simulink model "Model2"  (R2023b)
settings: Solver=ode4  StartTime=0.0  StopTime=50  FixedStep=0.01  RelTol=1e-3
values from neighbouring files (symbols this model uses):
  ARM_P_PID = [10 0 20]*0.1    [Single_ARM_Monte.m]    (also in main_starter.m)
  ARM_T_PID = [100 0 0]    [Single_ARM_Monte.m]    (also in main_starter.m)
  ARM_V_PID = [10 0 5]*0.1    [Single_ARM_Monte.m]    (also in main_starter.m)
  D = sqrt(px*px + py*py)    [test2.m]
  D_Joint0_angle0 = 45    [Single_ARM_Monte.m]    (also in main_starter.m)
  D_Joint0_angle1 = 0    [Single_ARM_Monte.m]    (also in main_starter.m)
  D_Joint0_angle2 = 0    [Single_ARM_Monte.m]    (also in main_starter.m)
  D_Joint0_rate0 = 0    [Single_ARM_Monte.m]    (also in main_starter.m)
  D_Joint0_rate1 = 0    [Single_ARM_Monte.m]    (also in main_starter.m)
  D_Joint0_rate2 = 0    [Single_ARM_Monte.m]    (also in main_starter.m)
  Joint_Motor_Mass = 23    [Single_ARM_Monte.m]    (also in main_starter.m)
  L_Joint0_angle0 = 45    [Single_ARM_Monte.m]    (also in main_starter.m)
  L_Joint0_angle1 = 0    [Single_ARM_Monte.m]    (also in main_starter.m)
  L_Joint0_angle2 = 0    [Single_ARM_Monte.m]    (also in main_starter.m)
  L_Joint0_rate0 = 0    [Single_ARM_Monte.m]    (also in main_starter.m)
  L_Joint0_rate1 = 0    [Single_ARM_Monte.m]    (also in main_starter.m)
  L_Joint0_rate2 = 0    [Single_ARM_Monte.m]    (also in main_starter.m)
  L_Joint_Offset = [ ... (first row only)    [Single_ARM_Monte.m]    (also in main_starter.m)
  Link1_Mass = 11    [Single_ARM_Monte.m]    (also in main_starter.m)
  Link2_Mass = 15.6    [Single_ARM_Monte.m]    (also in main_starter.m)
  Link3_Mass = 11    [Single_ARM_Monte.m]    (also in main_starter.m)
  Motor_transfer_Den = [1 100]    [Single_ARM_Monte.m]    (also in main_starter.m)
  Motor_transfer_Num = [100]    [Single_ARM_Monte.m]    (also in main_starter.m)
  PID_dt = 0.01    [Single_ARM_Monte.m]    (also in main_starter.m)
  R_Joint0_angle0 = 45    [Single_ARM_Monte.m]    (also in main_starter.m)
  R_Joint0_angle1 = 0    [Single_ARM_Monte.m]    (also in main_starter.m)
  R_Joint0_angle2 = 0    [Single_ARM_Monte.m]    (also in main_starter.m)
  R_Joint0_rate0 = 0    [Single_ARM_Monte.m]    (also in main_starter.m)
  R_Joint0_rate1 = 0    [Single_ARM_Monte.m]    (also in main_starter.m)
  R_Joint0_rate2 = 0    [Single_ARM_Monte.m]    (also in main_starter.m)
  RW_Att_D = 0.5    [Single_ARM_Monte.m]    (also in main_starter.m)
  RW_Att_I = 0.2    [Single_ARM_Monte.m]    (also in main_starter.m)
  RW_Att_P = 0.1    [Single_ARM_Monte.m]    (also in main_starter.m)
  RW_Mass = 100    [Single_ARM_Monte.m]    (also in main_starter.m)
  S_Body_Mass = 5    [Single_ARM_Monte.m]    (also in main_starter.m)
  S_init_pos = [0 0 0]'    [Single_ARM_Monte.m]    (also in main_starter.m)
  S_init_vel = [0 0 0]'    [Single_ARM_Monte.m]    (also in main_starter.m)
  T_Body_Mass = 4    [Single_ARM_Monte.m]    (also in main_starter.m)
  T_init_pos = [T_init_pos_list(i,1) T_init_pos_list(i,2) 0]'    [Single_ARM_Monte.m]    (also in main_starter.m = [0.3 0 0]')
  T_init_vel = [0 0 0]'    [Single_ARM_Monte.m]    (also in main_starter.m)
  Torq_mea_transfer_Den = [1 5]    [Single_ARM_Monte.m]    (also in main_starter.m)
  Torq_mea_transfer_Num = [5]    [Single_ARM_Monte.m]    (also in main_starter.m)
  U_Joint0_angle0 = 45    [Single_ARM_Monte.m]    (also in main_starter.m)
  U_Joint0_angle1 = 0    [Single_ARM_Monte.m]    (also in main_starter.m)
  U_Joint0_angle2 = 0    [Single_ARM_Monte.m]    (also in main_starter.m)
  U_Joint0_rate0 = 0    [Single_ARM_Monte.m]    (also in main_starter.m)
  U_Joint0_rate1 = 0    [Single_ARM_Monte.m]    (also in main_starter.m)
  U_Joint0_rate2 = 0    [Single_ARM_Monte.m]    (also in main_starter.m)
undefined symbols (not defined in the file or in its folder): X, Y, Z
libraries: nesl_utility x315, sm_lib x281, simulink_extras x48, sharedtransform x25, aerolibutil x4
(part 8 of 12)

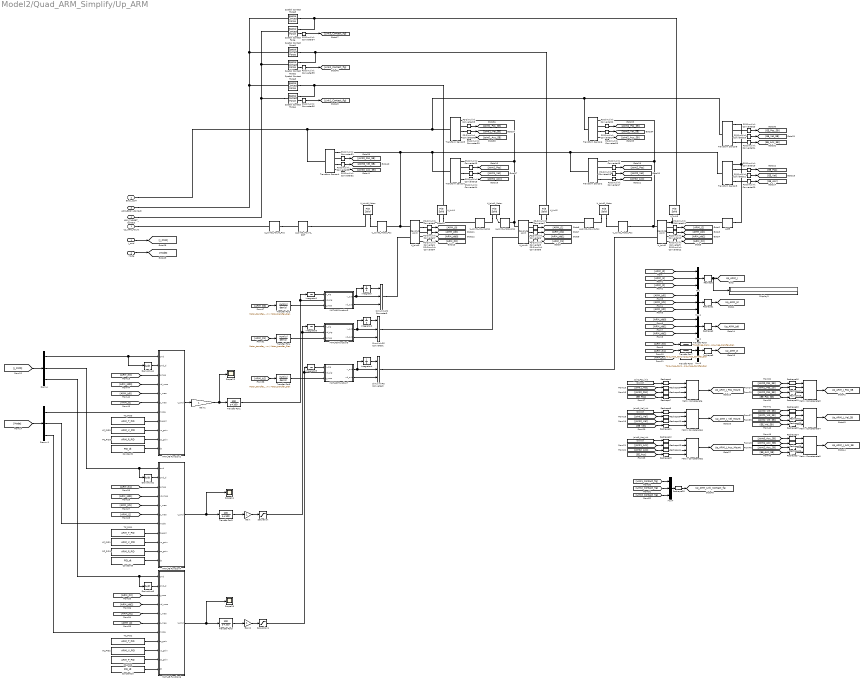
== system Model2/Quad_ARM_Simplify/Up_ARM ==
  J_cmd : Inport
  Mode : Inport  Port=2
  Constant10 : Constant  Value=PID_dt
  Constant2 : Constant  Value=PID_dt
  Constant9 : Constant  Value=PID_dt
  Demux : Demux  Outputs=3
  Demux1 : Demux  Outputs=3
  Derivative1 : Derivative
  Derivative2 : Derivative
  Derivative3 : Derivative
  Display3 : Display
  Gain : Gain
  Gain1 : Gain
  Gain2 : Gain
  Integrator : Integrator  InitialCondition=-U_Joint0_angle0*(pi/180)
  Integrator1 : Integrator  InitialCondition=-U_Joint0_rate0*(pi/180)
  Integrator2 : Integrator  InitialCondition=-U_Joint0_angle1*(pi/180)
  Integrator3 : Integrator  InitialCondition=-U_Joint0_rate1*(pi/180)
  Integrator4 : Integrator  InitialCondition=-U_Joint0_angle2*(pi/180)
  Integrator5 : Integrator  InitialCondition=-U_Joint0_rate2*(pi/180)
  Joint0_Acc_init : Constant  Value=[0 0 0]'
  Joint0_Vel_init : Constant  Value=[0 0 0]'
  Joint_Pos_init : Constant  Value=[0 0 0]'
  MATLAB Function2 : MATLAB Function  TreatAsAtomicUnit=on
  MATLAB Function3 : MATLAB Function  TreatAsAtomicUnit=on
  MATLAB Function4 : MATLAB Function  TreatAsAtomicUnit=on
  MATLAB Function5 : MATLAB Function  TreatAsAtomicUnit=on
  MATLAB Function6 : MATLAB Function  TreatAsAtomicUnit=on
  MATLAB Function7 : MATLAB Function  TreatAsAtomicUnit=on
  Matrix Concatenate{,1..5} (6 alike) : Concatenate  NumInputs=4  Mode=Multidimensional array  ConcatenateDimension=2
  Mux{,1..4} (5 alike) : Mux  Inputs=3
  PC_PID1 : Constant  Value=ARM_P_PID
  PC_PID2 : Constant  Value=ARM_P_PID
  PC_PID3 : Constant  Value=ARM_P_PID
  PS-Simulink Converter{1..36} (36 alike) : nesl_utility/PS-Simulink Converter  PhysicalDomain=network_engine_domain  SubClassName=ps_output  LeftPortType=input  RightPortType=output  PseudoPeriodic=off  Frequencies=[]  VectorFormat=inherit  Unit=inherit  AffineConversion=off
  Reshape{,1..28} (29 alike) : Reshape  OutputDimensionality=Column vector (2-D)
  Saturation : Saturate  UpperLimit=2  LowerLimit=-2
  Saturation1 : Saturate  UpperLimit=2  LowerLimit=-2
  Scope11 : Scope
  Scope13 : Scope
  Scope15 : Scope
  Simulink-PS Converter1 : nesl_utility/Simulink-PS Converter  PhysicalDomain=network_engine_domain  SubClassName=ps_input  LeftPortType=input  RightPortType=output  PseudoPeriodic=off  Frequencies=[]  NoiseDistribution=none  NoiseParameters=[]  Unit=1  AffineConversion=off  FilteringAndDerivatives=provide  SimscapeFilterOrder=1  InputFilterTimeConstant=0.001  UdotUserProvided=2
  Simulink-PS Converter2 : nesl_utility/Simulink-PS Converter  PhysicalDomain=network_engine_domain  SubClassName=ps_input  LeftPortType=input  RightPortType=output  PseudoPeriodic=off  Frequencies=[]  NoiseDistribution=none  NoiseParameters=[]  Unit=1  AffineConversion=off  FilteringAndDerivatives=provide  SimscapeFilterOrder=1  InputFilterTimeConstant=0.001  UdotUserProvided=2
  Simulink-PS Converter9 : nesl_utility/Simulink-PS Converter  PhysicalDomain=network_engine_domain  SubClassName=ps_input  LeftPortType=input  RightPortType=output  PseudoPeriodic=off  Frequencies=[]  NoiseDistribution=none  NoiseParameters=[]  Unit=1  AffineConversion=off  FilteringAndDerivatives=provide  SimscapeFilterOrder=1  InputFilterTimeConstant=0.001  UdotUserProvided=2
  Spatial Contact Force : sm_lib/Forces and Torques/Spatial Contact Force  SenseContactBaseRotation=off  SenseContactBaseTranslation=off  CoefficientOfDynamicFriction=L2T_DF  CoefficientOfStaticFriction=L2T_SF  NormalDamping=L32T_Damping  NormalDampingUnits=N/(m/s)  SenseContactSignal=on  NormalStiffness=L32T_Siffness  NormalStiffnessUnits=N/m  FrictionalCriticalVelocity=L2T_CV  FrictionalCriticalVelocityUnits=m/s  ZeroCrossDetectContactStartAndEnd=off  SenseContactFollowerRotation=off  SenseContactFollowerTranslation=off  FrictionType=SmoothStickSlip  SenseFrictionalForceMagnitude=off  SenseNormalForceMagnitude=off  NormalForceType=SmoothSpringDamper  SenseNormalVelocity=off  SensePenetrationDepth=off  SenseSeparationDistance=off  SenseTangentialVelocity=off  NormalTransitionRegionWidth=L32T_TRW  NormalTransitionRegionWidthUnits=m
  Spatial Contact Force1 : sm_lib/Forces and Torques/Spatial Contact Force  SenseContactBaseRotation=off  SenseContactBaseTranslation=off  CoefficientOfDynamicFriction=L2B_DF  CoefficientOfStaticFriction=L2B_SF  NormalDamping=L22B_Damping  NormalDampingUnits=N/(m/s)  SenseContactSignal=off  NormalStiffness=L22B_Stiffness  NormalStiffnessUnits=N/m  FrictionalCriticalVelocity=L2B_CV  FrictionalCriticalVelocityUnits=m/s  ZeroCrossDetectContactStartAndEnd=off  SenseContactFollowerRotation=off  SenseContactFollowerTranslation=off  FrictionType=SmoothStickSlip  SenseFrictionalForceMagnitude=off  SenseNormalForceMagnitude=off  NormalForceType=SmoothSpringDamper  SenseNormalVelocity=off  SensePenetrationDepth=off  SenseSeparationDistance=off  SenseTangentialVelocity=off  NormalTransitionRegionWidth=L22B_TRW  NormalTransitionRegionWidthUnits=m
  Spatial Contact Force2 : sm_lib/Forces and Torques/Spatial Contact Force  SenseContactBaseRotation=off  SenseContactBaseTranslation=off  CoefficientOfDynamicFriction=L2T_DF  CoefficientOfStaticFriction=L2T_SF  NormalDamping=L22T_Damping  NormalDampingUnits=N/(m/s)  SenseContactSignal=on  NormalStiffness=L22T_Siffness  NormalStiffnessUnits=N/m  FrictionalCriticalVelocity=L2T_CV  FrictionalCriticalVelocityUnits=m/s  ZeroCrossDetectContactStartAndEnd=off  SenseContactFollowerRotation=off  SenseContactFollowerTranslation=off  FrictionType=SmoothStickSlip  SenseFrictionalForceMagnitude=off  SenseNormalForceMagnitude=off  NormalForceType=SmoothSpringDamper  SenseNormalVelocity=off  SensePenetrationDepth=off  SenseSeparationDistance=off  SenseTangentialVelocity=off  NormalTransitionRegionWidth=L22T_TRW  NormalTransitionRegionWidthUnits=m
  Spatial Contact Force3 : sm_lib/Forces and Torques/Spatial Contact Force  SenseContactBaseRotation=off  SenseContactBaseTranslation=off  CoefficientOfDynamicFriction=L2B_DF  CoefficientOfStaticFriction=L2B_SF  NormalDamping=L12B_Damping  NormalDampingUnits=N/(m/s)  SenseContactSignal=off  NormalStiffness=L12B_Stiffness  NormalStiffnessUnits=N/m  FrictionalCriticalVelocity=L2B_CV  FrictionalCriticalVelocityUnits=m/s  ZeroCrossDetectContactStartAndEnd=off  SenseContactFollowerRotation=off  SenseContactFollowerTranslation=off  FrictionType=SmoothStickSlip  SenseFrictionalForceMagnitude=off  SenseNormalForceMagnitude=off  NormalForceType=SmoothSpringDamper  SenseNormalVelocity=off  SensePenetrationDepth=off  SenseSeparationDistance=off  SenseTangentialVelocity=off  NormalTransitionRegionWidth=L12B_TRW  NormalTransitionRegionWidthUnits=m
  Spatial Contact Force4 : sm_lib/Forces and Torques/Spatial Contact Force  SenseContactBaseRotation=off  SenseContactBaseTranslation=off  CoefficientOfDynamicFriction=L2T_DF  CoefficientOfStaticFriction=L2T_SF  NormalDamping=L12T_Damping  NormalDampingUnits=N/(m/s)  SenseContactSignal=on  NormalStiffness=L12T_Siffness  NormalStiffnessUnits=N/m  FrictionalCriticalVelocity=L2T_CV  FrictionalCriticalVelocityUnits=m/s  ZeroCrossDetectContactStartAndEnd=off  SenseContactFollowerRotation=off  SenseContactFollowerTranslation=off  FrictionType=SmoothStickSlip  SenseFrictionalForceMagnitude=off  SenseNormalForceMagnitude=off  NormalForceType=SmoothSpringDamper  SenseNormalVelocity=off  SensePenetrationDepth=off  SenseSeparationDistance=off  SenseTangentialVelocity=off  NormalTransitionRegionWidth=L12T_TRW  NormalTransitionRegionWidthUnits=m
  Spatial Contact Force5 : sm_lib/Forces and Torques/Spatial Contact Force  SenseContactBaseRotation=off  SenseContactBaseTranslation=off  CoefficientOfDynamicFriction=L2B_DF  CoefficientOfStaticFriction=L2B_SF  NormalDamping=L32B_Damping  NormalDampingUnits=N/(m/s)  SenseContactSignal=off  NormalStiffness=L32B_Stiffness  NormalStiffnessUnits=N/m  FrictionalCriticalVelocity=L2B_CV  FrictionalCriticalVelocityUnits=m/s  ZeroCrossDetectContactStartAndEnd=off  SenseContactFollowerRotation=off  SenseContactFollowerTranslation=off  FrictionType=SmoothStickSlip  SenseFrictionalForceMagnitude=off  SenseNormalForceMagnitude=off  NormalForceType=SmoothSpringDamper  SenseNormalVelocity=off  SensePenetrationDepth=off  SenseSeparationDistance=off  SenseTangentialVelocity=off  NormalTransitionRegionWidth=L32B_TRW  NormalTransitionRegionWidthUnits=m
  TC_PID1 : Constant  Value=ARM_T_PID
  TC_PID2 : Constant  Value=ARM_T_PID
  TC_PID3 : Constant  Value=ARM_T_PID
  Transfer Fcn1 : TransferFcn  Numerator=[100]  Denominator=[1 100]
  Transfer Fcn2 : TransferFcn  Numerator=Motor_transfer_Num  Denominator=Motor_transfer_Den
  Transfer Fcn3 : TransferFcn  Numerator=[100]  Denominator=[1 100]
  Transfer Fcn4 : TransferFcn  Numerator=Motor_transfer_Num  Denominator=Motor_transfer_Den
  Transfer Fcn5 : TransferFcn  Numerator=[100]  Denominator=[1 100]
  Transfer Fcn6 : TransferFcn  Numerator=Motor_transfer_Num  Denominator=Motor_transfer_Den
  Transfer Fcn7 : TransferFcn  Numerator=Torq_mea_transfer_Num  Denominator=Torq_mea_transfer_Den
  Transfer Fcn8 : TransferFcn  Numerator=Torq_mea_transfer_Num  Denominator=Torq_mea_transfer_Den
  Transfer Fcn9 : TransferFcn  Numerator=Torq_mea_transfer_Num  Denominator=Torq_mea_transfer_Den
  Transform Sensor{1..6,8} (7 alike) : sm_lib/Frames and Transforms/Transform Sensor  MeasurementFrame=Base  RotationSequence=ZYX  SenseAngle=off  SenseAxis=off  SenseQ=off  SenseR=off  SenseRotationSequence=off  SenseOmegaX=off  SenseOmegaY=off  SenseOmegaZ=off  SenseOmega=off  SenseQDot=off  SenseRDot=off  SenseRotationSequenceDot=off  SenseAlphaX=off  SenseAlphaY=off  SenseAlphaZ=off  SenseAlpha=off  SenseQDDot=off  SenseRDDot=off  SenseX=off  SenseY=off  SenseZ=off  SenseXYZ=on  SenseRad=off  SenseAzim=off  SenseDist=off  SenseInc=off  SenseXDot=off  SenseYDot=off  SenseZDot=off  SenseXYZDot=on  SenseRadDot=off  SenseAzimDot=off  SenseDistDot=off  SenseIncDot=off  SenseXDDot=off  SenseYDDot=off  SenseZDDot=off  SenseXYZDDot=on  SenseRadDDot=off  SenseAzimDDot=off  SenseDistDDot=off  SenseIncDDot=off
  U_EE : sm_lib/Frames and Transforms/Rigid Transform  TranslationMethod=Cartesian  TranslationStandardOffset=0  TranslationStandardOffsetUnits=m  TranslationStandardAxis=+Z  TranslationCartesianOffset=[12.315 2.945 0]  TranslationCartesianOffsetUnits=cm  TranslationROffset=0  TranslationROffsetUnits=m  TranslationZOffset=0  TranslationZOffsetUnits=m  TranslationThetaOffset=0  TranslationThetaOffsetUnits=deg  RotationMethod=None  RotationAngleUnits=deg  RotationStandardAxis=+Z  RotationAngle=0.0  RotationArbitraryAxis=[0 0 1]  FollAlignAxisA=+X  BaseAlignAxisA=+Y  FollAlignAxisB=+Y  BaseAlignAxisB=+Z  RotationSequenceAxes=FollowerAxes  RotationSequence=ZYX  RotationSequenceAngles=[0 0 0]  RotationSequenceAnglesUnits=deg  RotationMatrix=[1 0 0; 0 1 0; 0 0 1]  Quaternion=[1 0 0 0]
  U_Joint0 : sm_lib/Joints/Revolute Joint  JointMode=Normal  SenseConstraintForce=off  SenseConstraintForceX=off  SenseConstraintForceY=off  SenseConstraintForceZ=off  SenseConstraintTorque=off  SenseConstraintTorqueX=off  SenseConstraintTorqueY=off  SenseConstraintTorqueZ=off  SenseTotalForce=off  SenseTotalForceX=off  SenseTotalForceY=off  SenseTotalForceZ=off  SenseTotalTorque=off  SenseTotalTorqueX=off  SenseTotalTorqueY=off  SenseTotalTorqueZ=off  CompositeWrenchDir=FollowerOnBase  CompositeWrenchFrame=BaseFrame  EquilibriumPosition=0  EquilibriumPositionUnits=deg  SpringStiffness=0  SpringStiffnessUnits=N*m/deg  DampingCoefficient=0  DampingCoefficientUnits=N*m/(deg/s)  TorqueActuationMode=ComputedTorque  MotionActuationMode=InputMotion  SensePosition=on  SenseVelocity=on  SenseAcceleration=on  SenseTorqueForce=on  SenseLowerLimitTorqueForce=off  SenseUpperLimitTorqueForce=off  LowerLimitSpecify=off  LowerLimitBound=-90  LowerLimitBoundUnits=deg  LowerLimitStiffness=1e4  LowerLimitStiffnessUnits=N*m/deg  LowerLimitDamping=1000  LowerLimitDampingUnits=N*m/(deg/s)  LowerLimitTransitionRegionWidth=0.1  LowerLimitTransitionRegionWidthUnits=deg  UpperLimitSpecify=off  UpperLimitBound=90  UpperLimitBoundUnits=deg  UpperLimitStiffness=1e4  UpperLimitStiffnessUnits=N*m/deg  UpperLimitDamping=1000  UpperLimitDampingUnits=N*m/(deg/s)  UpperLimitTransitionRegionWidth=0.1  UpperLimitTransitionRegionWidthUnits=deg  PositionTargetSpecify=on  PositionTargetPriority=High  PositionTargetValue=-U_Joint0_angle0  PositionTargetValueUnits=deg  VelocityTargetSpecify=on  VelocityTargetPriority=High  VelocityTargetValue=-U_Joint0_rate0  VelocityTargetValueUnits=deg/s
  U_Joint0_Motor : sm_lib/Body Elements/File Solid  ExtGeomFileName=..\Joint_Motor\XL_XC-330.stp  UnitType=Custom  ExtGeomFileUnits=mm  StepReaderType=HEX  ExportConvexHullGeometry=off  InertiaType=CalculateFromGeometry  Mass=Joint_Motor_Mass  MassUnits=g  CenterOfMass=[0 0 0]  CenterOfMassUnits=m  MomentsOfInertia=[1 1 1]  MomentsOfInertiaUnits=kg*m^2  ProductsOfInertia=[0 0 0]  ProductsOfInertiaUnits=kg*m^2  BasedOnType=Mass  Density=1000  DensityUnits=kg/m^3  DoExposeReferenceFrame=on  SerializedFrames=<Frames><Frame><Id>Frame1</Id><Value><Name>Mount_F</Name><Origin><Source>CenterOfMassFrame</Source><FeatureName></FeatureName></Origin><PrimaryAxis><DefinedDirection>+Z</DefinedDirection><Source>ReferenceFrame</Source><SourceDirection>+Z</SourceDirection><FeatureName></FeatureName></PrimaryAxis><SecondaryAxis><DefinedDirection>+X</DefinedDirection><Source>ReferenceFrame</Source><SourceDirection>+Y</SourceDirection><FeatureName></FeatureName></SecondaryAxis></Value></Frame><Frame><Id>Frame2</Id><Value><Name>CoM_F</Name><Origin><Source>CenterOfMassFrame</Source><FeatureName></FeatureName></Origin><PrimaryAxis><DefinedDirection>+Z</DefinedDirection><Source>ReferenceFrame</Source><SourceDirection>+Z</SourceDirection><FeatureName></FeatureName></PrimaryAxis><SecondaryAxis><DefinedDirection>+X</DefinedDirection><Source>ReferenceFrame</Source><SourceDirection>+Y</SourceDirection><FeatureName></FeatureName></SecondaryAxis></Value></Frame></Frames>  GraphicType=FromGeometry  MarkerShape=Sphere  MarkerSize=10  GraphicVisPropType=SimpleVisualProperties  GraphicDiffuseColor=[0.4 0.4 0.4]  GraphicSpecularColor=[0.5 0.5 0.5 1.0]  GraphicAmbientColor=[0.15 0.15 0.15 1.0]  GraphicEmissiveColor=[0.0 0.0 0.0 1.0]  GraphicShininess=75  GraphicOpacity=1.0
  U_Joint0_Motor_Pos : sm_lib/Frames and Transforms/Rigid Transform  TranslationMethod=Cartesian  TranslationStandardOffset=0  TranslationStandardOffsetUnits=m  TranslationStandardAxis=+Z  TranslationCartesianOffset=[0.69 0 0]  TranslationCartesianOffsetUnits=cm  TranslationROffset=0  TranslationROffsetUnits=m  TranslationZOffset=0  TranslationZOffsetUnits=m  TranslationThetaOffset=0  TranslationThetaOffsetUnits=deg  RotationMethod=None  RotationAngleUnits=deg  RotationStandardAxis=+Z  RotationAngle=0.0  RotationArbitraryAxis=[0 0 1]  FollAlignAxisA=+X  BaseAlignAxisA=+Y  FollAlignAxisB=+Y  BaseAlignAxisB=+Z  RotationSequenceAxes=FollowerAxes  RotationSequence=ZYX  RotationSequenceAngles=[-90 0 0]  RotationSequenceAnglesUnits=deg  RotationMatrix=[1 0 0; 0 1 0; 0 0 1]  Quaternion=[1 0 0 0]
  U_Joint0_Mount_Pos : sm_lib/Frames and Transforms/Rigid Transform  TranslationMethod=Cartesian  TranslationStandardOffset=0  TranslationStandardOffsetUnits=m  TranslationStandardAxis=+Z  TranslationCartesianOffset=[8.35+2.5 0 (19.7+2.5)]  TranslationCartesianOffsetUnits=cm  TranslationROffset=0  TranslationROffsetUnits=m  TranslationZOffset=0  TranslationZOffsetUnits=m  TranslationThetaOffset=0  TranslationThetaOffsetUnits=deg  RotationMethod=None  RotationAngleUnits=deg  RotationStandardAxis=+Z  RotationAngle=0.0  RotationArbitraryAxis=[0 0 1]  FollAlignAxisA=+X  BaseAlignAxisA=+Y  FollAlignAxisB=+Y  BaseAlignAxisB=+Z  RotationSequenceAxes=FollowerAxes  RotationSequence=XYX  RotationSequenceAngles=[0 0 0]  RotationSequenceAnglesUnits=deg  RotationMatrix=[1 0 0; 0 1 0; 0 0 1]  Quaternion=[1 0 0 0]
  U_Joint0_Mount_ROT : sm_lib/Frames and Transforms/Rigid Transform  TranslationMethod=None  TranslationStandardOffset=0  TranslationStandardOffsetUnits=m  TranslationStandardAxis=+Z  TranslationCartesianOffset=[8.35+2.5 -(14.7+2.5) 0]  TranslationCartesianOffsetUnits=cm  TranslationROffset=0  TranslationROffsetUnits=m  TranslationZOffset=0  TranslationZOffsetUnits=m  TranslationThetaOffset=0  TranslationThetaOffsetUnits=deg  RotationMethod=RotationSequence  RotationAngleUnits=deg  RotationStandardAxis=+Z  RotationAngle=0.0  RotationArbitraryAxis=[0 0 1]  FollAlignAxisA=+X  BaseAlignAxisA=+Y  FollAlignAxisB=+Y  BaseAlignAxisB=+Z  RotationSequenceAxes=FollowerAxes  RotationSequence=ZYX  RotationSequenceAngles=[0 0 -90]  RotationSequenceAnglesUnits=deg  RotationMatrix=[1 0 0; 0 1 0; 0 0 1]  Quaternion=[1 0 0 0]
  U_Joint1 : sm_lib/Joints/Revolute Joint  JointMode=Normal  SenseConstraintForce=off  SenseConstraintForceX=off  SenseConstraintForceY=off  SenseConstraintForceZ=off  SenseConstraintTorque=off  SenseConstraintTorqueX=off  SenseConstraintTorqueY=off  SenseConstraintTorqueZ=off  SenseTotalForce=off  SenseTotalForceX=off  SenseTotalForceY=off  SenseTotalForceZ=off  SenseTotalTorque=off  SenseTotalTorqueX=off  SenseTotalTorqueY=off  SenseTotalTorqueZ=off  CompositeWrenchDir=FollowerOnBase  CompositeWrenchFrame=BaseFrame  EquilibriumPosition=0  EquilibriumPositionUnits=deg  SpringStiffness=0  SpringStiffnessUnits=N*m/deg  DampingCoefficient=0  DampingCoefficientUnits=N*m/(deg/s)  TorqueActuationMode=ComputedTorque  MotionActuationMode=InputMotion  SensePosition=on  SenseVelocity=on  SenseAcceleration=on  SenseTorqueForce=on  SenseLowerLimitTorqueForce=off  SenseUpperLimitTorqueForce=off  LowerLimitSpecify=off  LowerLimitBound=-90  LowerLimitBoundUnits=deg  LowerLimitStiffness=1e4  LowerLimitStiffnessUnits=N*m/deg  LowerLimitDamping=10  LowerLimitDampingUnits=N*m/(deg/s)  LowerLimitTransitionRegionWidth=0.1  LowerLimitTransitionRegionWidthUnits=deg  UpperLimitSpecify=off  UpperLimitBound=90  UpperLimitBoundUnits=deg  UpperLimitStiffness=1e4  UpperLimitStiffnessUnits=N*m/deg  UpperLimitDamping=10  UpperLimitDampingUnits=N*m/(deg/s)  UpperLimitTransitionRegionWidth=0.1  UpperLimitTransitionRegionWidthUnits=deg  PositionTargetSpecify=on  PositionTargetPriority=High  PositionTargetValue=-U_Joint0_angle1  PositionTargetValueUnits=deg  VelocityTargetSpecify=on  VelocityTargetPriority=High  VelocityTargetValue=-U_Joint0_rate1  VelocityTargetValueUnits=deg/s
  U_Joint1_Motor : sm_lib/Body Elements/File Solid  ExtGeomFileName=..\Joint_Motor\XL_XC-330.stp  UnitType=Custom  ExtGeomFileUnits=mm  StepReaderType=HEX  ExportConvexHullGeometry=off  InertiaType=CalculateFromGeometry  Mass=Joint_Motor_Mass  MassUnits=g  CenterOfMass=[0 0 0]  CenterOfMassUnits=m  MomentsOfInertia=[1 1 1]  MomentsOfInertiaUnits=kg*m^2  ProductsOfInertia=[0 0 0]  ProductsOfInertiaUnits=kg*m^2  BasedOnType=Mass  Density=1000  DensityUnits=kg/m^3  DoExposeReferenceFrame=on  SerializedFrames=<Frames><Frame><Id>Frame1</Id><Value><Name>Mount_F</Name><Origin><Source>CenterOfMassFrame</Source><FeatureName></FeatureName></Origin><PrimaryAxis><DefinedDirection>+Z</DefinedDirection><Source>ReferenceFrame</Source><SourceDirection>+Z</SourceDirection><FeatureName></FeatureName></PrimaryAxis><SecondaryAxis><DefinedDirection>+X</DefinedDirection><Source>ReferenceFrame</Source><SourceDirection>+Y</SourceDirection><FeatureName></FeatureName></SecondaryAxis></Value></Frame><Frame><Id>Frame2</Id><Value><Name>CoM_F</Name><Origin><Source>CenterOfMassFrame</Source><FeatureName></FeatureName></Origin><PrimaryAxis><DefinedDirection>+Z</DefinedDirection><Source>ReferenceFrame</Source><SourceDirection>+Z</SourceDirection><FeatureName></FeatureName></PrimaryAxis><SecondaryAxis><DefinedDirection>+X</DefinedDirection><Source>ReferenceFrame</Source><SourceDirection>+Y</SourceDirection><FeatureName></FeatureName></SecondaryAxis></Value></Frame></Frames>  GraphicType=FromGeometry  MarkerShape=Sphere  MarkerSize=10  GraphicVisPropType=SimpleVisualProperties  GraphicDiffuseColor=[0.4 0.4 0.4]  GraphicSpecularColor=[0.5 0.5 0.5 1.0]  GraphicAmbientColor=[0.15 0.15 0.15 1.0]  GraphicEmissiveColor=[0.0 0.0 0.0 1.0]  GraphicShininess=75  GraphicOpacity=1.0
  U_Joint1_Motor_Pos : sm_lib/Frames and Transforms/Rigid Transform  TranslationMethod=Cartesian  TranslationStandardOffset=0  TranslationStandardOffsetUnits=m  TranslationStandardAxis=+Z  TranslationCartesianOffset=[0.685 0 0]  TranslationCartesianOffsetUnits=cm  TranslationROffset=0  TranslationROffsetUnits=m  TranslationZOffset=0  TranslationZOffsetUnits=m  TranslationThetaOffset=0  TranslationThetaOffsetUnits=deg  RotationMethod=None  RotationAngleUnits=deg  RotationStandardAxis=+Z  RotationAngle=0.0  RotationArbitraryAxis=[0 0 1]  FollAlignAxisA=+X  BaseAlignAxisA=+Y  FollAlignAxisB=+Y  BaseAlignAxisB=+Z  RotationSequenceAxes=FollowerAxes  RotationSequence=ZYX  RotationSequenceAngles=[-90 0 0]  RotationSequenceAnglesUnits=deg  RotationMatrix=[1 0 0; 0 1 0; 0 0 1]  Quaternion=[1 0 0 0]
  U_Joint1_Mount_Pos : sm_lib/Frames and Transforms/Rigid Transform  TranslationMethod=Cartesian  TranslationStandardOffset=0  TranslationStandardOffsetUnits=m  TranslationStandardAxis=+Z  TranslationCartesianOffset="[5.94 -0.75  0]"  TranslationCartesianOffsetUnits=cm  TranslationROffset=0  TranslationROffsetUnits=m  TranslationZOffset=0  TranslationZOffsetUnits=m  TranslationThetaOffset=0  TranslationThetaOffsetUnits=deg  RotationMethod=None  RotationAngleUnits=deg  RotationStandardAxis=+Z  RotationAngle=0.0  RotationArbitraryAxis=[0 0 1]  FollAlignAxisA=+X  BaseAlignAxisA=+Y  FollAlignAxisB=+Y  BaseAlignAxisB=+Z  RotationSequenceAxes=FollowerAxes  RotationSequence=ZYX  RotationSequenceAngles=[-90 0 0]  RotationSequenceAnglesUnits=deg  RotationMatrix=[1 0 0; 0 1 0; 0 0 1]  Quaternion=[1 0 0 0]
  U_Joint2 : sm_lib/Joints/Revolute Joint  JointMode=Normal  SenseConstraintForce=off  SenseConstraintForceX=off  SenseConstraintForceY=off  SenseConstraintForceZ=off  SenseConstraintTorque=off  SenseConstraintTorqueX=off  SenseConstraintTorqueY=off  SenseConstraintTorqueZ=off  SenseTotalForce=off  SenseTotalForceX=off  SenseTotalForceY=off  SenseTotalForceZ=off  SenseTotalTorque=off  SenseTotalTorqueX=off  SenseTotalTorqueY=off  SenseTotalTorqueZ=off  CompositeWrenchDir=FollowerOnBase  CompositeWrenchFrame=BaseFrame  EquilibriumPosition=0  EquilibriumPositionUnits=deg  SpringStiffness=0  SpringStiffnessUnits=N*m/deg  DampingCoefficient=0  DampingCoefficientUnits=N*m/(deg/s)  TorqueActuationMode=ComputedTorque  MotionActuationMode=InputMotion  SensePosition=on  SenseVelocity=on  SenseAcceleration=on  SenseTorqueForce=on  SenseLowerLimitTorqueForce=off  SenseUpperLimitTorqueForce=off  LowerLimitSpecify=off  LowerLimitBound=-90  LowerLimitBoundUnits=deg  LowerLimitStiffness=1e4  LowerLimitStiffnessUnits=N*m/deg  LowerLimitDamping=10  LowerLimitDampingUnits=N*m/(deg/s)  LowerLimitTransitionRegionWidth=0.1  LowerLimitTransitionRegionWidthUnits=deg  UpperLimitSpecify=off  UpperLimitBound=90  UpperLimitBoundUnits=deg  UpperLimitStiffness=1e4  UpperLimitStiffnessUnits=N*m/deg  UpperLimitDamping=10  UpperLimitDampingUnits=N*m/(deg/s)  UpperLimitTransitionRegionWidth=0.1  UpperLimitTransitionRegionWidthUnits=deg  PositionTargetSpecify=on  PositionTargetPriority=High  PositionTargetValue=-U_Joint0_angle2  PositionTargetValueUnits=deg  VelocityTargetSpecify=on  VelocityTargetPriority=High  VelocityTargetValue=-U_Joint0_rate2  VelocityTargetValueUnits=deg/s
  U_Joint2_Motor : sm_lib/Body Elements/File Solid  ExtGeomFileName=..\Joint_Motor\XL_XC-330.stp  UnitType=Custom  ExtGeomFileUnits=mm  StepReaderType=HEX  ExportConvexHullGeometry=off  InertiaType=CalculateFromGeometry  Mass=Joint_Motor_Mass  MassUnits=g  CenterOfMass=[0 0 0]  CenterOfMassUnits=m  MomentsOfInertia=[1 1 1]  MomentsOfInertiaUnits=kg*m^2  ProductsOfInertia=[0 0 0]  ProductsOfInertiaUnits=kg*m^2  BasedOnType=Mass  Density=1000  DensityUnits=kg/m^3  DoExposeReferenceFrame=on  SerializedFrames=<Frames><Frame><Id>Frame1</Id><Value><Name>Mount_F</Name><Origin><Source>CenterOfMassFrame</Source><FeatureName></FeatureName></Origin><PrimaryAxis><DefinedDirection>+Z</DefinedDirection><Source>ReferenceFrame</Source><SourceDirection>+Z</SourceDirection><FeatureName></FeatureName></PrimaryAxis><SecondaryAxis><DefinedDirection>+X</DefinedDirection><Source>ReferenceFrame</Source><SourceDirection>+Y</SourceDirection><FeatureName></FeatureName></SecondaryAxis></Value></Frame><Frame><Id>Frame2</Id><Value><Name>CoM_F</Name><Origin><Source>CenterOfMassFrame</Source><FeatureName></FeatureName></Origin><PrimaryAxis><DefinedDirection>+Z</DefinedDirection><Source>ReferenceFrame</Source><SourceDirection>+Z</SourceDirection><FeatureName></FeatureName></PrimaryAxis><SecondaryAxis><DefinedDirection>+X</DefinedDirection><Source>ReferenceFrame</Source><SourceDirection>+Y</SourceDirection><FeatureName></FeatureName></SecondaryAxis></Value></Frame></Frames>  GraphicType=FromGeometry  MarkerShape=Sphere  MarkerSize=10  GraphicVisPropType=SimpleVisualProperties  GraphicDiffuseColor=[0.4 0.4 0.4]  GraphicSpecularColor=[0.5 0.5 0.5 1.0]  GraphicAmbientColor=[0.15 0.15 0.15 1.0]  GraphicEmissiveColor=[0.0 0.0 0.0 1.0]  GraphicShininess=75  GraphicOpacity=1.0
  U_Joint2_Motor_Pos : sm_lib/Frames and Transforms/Rigid Transform  TranslationMethod=Cartesian  TranslationStandardOffset=0  TranslationStandardOffsetUnits=m  TranslationStandardAxis=+Z  TranslationCartesianOffset=[0.685 0 0]  TranslationCartesianOffsetUnits=cm  TranslationROffset=0  TranslationROffsetUnits=m  TranslationZOffset=0  TranslationZOffsetUnits=m  TranslationThetaOffset=0  TranslationThetaOffsetUnits=deg  RotationMethod=None  RotationAngleUnits=deg  RotationStandardAxis=+Z  RotationAngle=0.0  RotationArbitraryAxis=[0 0 1]  FollAlignAxisA=+X  BaseAlignAxisA=+Y  FollAlignAxisB=+Y  BaseAlignAxisB=+Z  RotationSequenceAxes=FollowerAxes  RotationSequence=ZYX  RotationSequenceAngles=[-90 0 0]  RotationSequenceAnglesUnits=deg  RotationMatrix=[1 0 0; 0 1 0; 0 0 1]  Quaternion=[1 0 0 0]
  U_Joint2_Mount_Pos : sm_lib/Frames and Transforms/Rigid Transform  TranslationMethod=Cartesian  TranslationStandardOffset=0  TranslationStandardOffsetUnits=m  TranslationStandardAxis=+Z  TranslationCartesianOffset=[8.67 0 0]  TranslationCartesianOffsetUnits=cm  TranslationROffset=0  TranslationROffsetUnits=m  TranslationZOffset=0  TranslationZOffsetUnits=m  TranslationThetaOffset=0  TranslationThetaOffsetUnits=deg  RotationMethod=None  RotationAngleUnits=deg  RotationStandardAxis=+Z  RotationAngle=0.0  RotationArbitraryAxis=[0 0 1]  FollAlignAxisA=+X  BaseAlignAxisA=+Y  FollAlignAxisB=+Y  BaseAlignAxisB=+Z  RotationSequenceAxes=FollowerAxes  RotationSequence=ZYX  RotationSequenceAngles=[-90 0 0]  RotationSequenceAnglesUnits=deg  RotationMatrix=[1 0 0; 0 1 0; 0 0 1]  Quaternion=[1 0 0 0]
  U_Link1 : sm_lib/Body Elements/File Solid  ExtGeomFileName=..\Right_ARM\Link_1_right.stp  UnitType=Custom  ExtGeomFileUnits=mm  StepReaderType=HEX  ExportConvexHullGeometry=on  InertiaType=CalculateFromGeometry  Mass=Link1_Mass  MassUnits=g  CenterOfMass=[0 0 0]  CenterOfMassUnits=m  MomentsOfInertia=[1 1 1]  MomentsOfInertiaUnits=kg*m^2  ProductsOfInertia=[0 0 0]  ProductsOfInertiaUnits=kg*m^2  BasedOnType=Mass  Density=1000  DensityUnits=kg/m^3  DoExposeReferenceFrame=on  SerializedFrames=<Frames><Frame><Id>Frame1</Id><Value><Name>Mount_F</Name><Origin><Source>ReferenceFrame</Source><FeatureName></FeatureName></Origin><PrimaryAxis><DefinedDirection>+Z</DefinedDirection><Source>ReferenceFrame</Source><SourceDirection>+Z</SourceDirection><FeatureName></FeatureName></PrimaryAxis><SecondaryAxis><DefinedDirection>+X</DefinedDirection><Source>ReferenceFrame</Source><SourceDirection>+Y</SourceDirection><FeatureName></FeatureName></SecondaryAxis></Value></Frame><Frame><Id>Frame2</Id><Value><Name>Joint_F</Name><Origin><Source>CenterOfMassFrame</Source><FeatureName></FeatureName></Origin><PrimaryAxis><DefinedDirection>+Z</DefinedDirection><Source>ReferenceFrame</Source><SourceDirection>+Z</SourceDirection><FeatureName></FeatureName></PrimaryAxis><SecondaryAxis><DefinedDirection>+X</DefinedDirection><Source>ReferenceFrame</Source><SourceDirection>+Y</SourceDirection><FeatureName></FeatureName></SecondaryAxis></Value></Frame></Frames>  GraphicType=FromGeometry  MarkerShape=Sphere  MarkerSize=10  GraphicVisPropType=SimpleVisualProperties  GraphicDiffuseColor=[0.0 0.2 1.0]  GraphicSpecularColor=[0.5 0.5 0.5 1.0]  GraphicAmbientColor=[0.15 0.15 0.15 1.0]  GraphicEmissiveColor=[0.0 0.0 0.0 1.0]  GraphicShininess=75  GraphicOpacity=1.0
  U_Link2 : sm_lib/Body Elements/File Solid  ExtGeomFileName=..\Right_ARM\Link_2_right.stp  UnitType=Custom  ExtGeomFileUnits=mm  StepReaderType=HEX  ExportConvexHullGeometry=on  InertiaType=CalculateFromGeometry  Mass=Link2_Mass  MassUnits=g  CenterOfMass=[0 0 0]  CenterOfMassUnits=m  MomentsOfInertia=[1 1 1]  MomentsOfInertiaUnits=kg*m^2  ProductsOfInertia=[0 0 0]  ProductsOfInertiaUnits=kg*m^2  BasedOnType=Mass  Density=1000  DensityUnits=kg/m^3  DoExposeReferenceFrame=on  SerializedFrames=<Frames><Frame><Id>Frame1</Id><Value><Name>Mount_F</Name><Origin><Source>ReferenceFrame</Source><FeatureName></FeatureName></Origin><PrimaryAxis><DefinedDirection>+Z</DefinedDirection><Source>ReferenceFrame</Source><SourceDirection>+Z</SourceDirection><FeatureName></FeatureName></PrimaryAxis><SecondaryAxis><DefinedDirection>+X</DefinedDirection><Source>ReferenceFrame</Source><SourceDirection>+Y</SourceDirection><FeatureName></FeatureName></SecondaryAxis></Value></Frame><Frame><Id>Frame2</Id><Value><Name>Joint_F</Name><Origin><Source>CenterOfMassFrame</Source><FeatureName></FeatureName></Origin><PrimaryAxis><DefinedDirection>+Z</DefinedDirection><Source>ReferenceFrame</Source><SourceDirection>+Z</SourceDirection><FeatureName></FeatureName></PrimaryAxis><SecondaryAxis><DefinedDirection>+X</DefinedDirection><Source>ReferenceFrame</Source><SourceDirection>+Y</SourceDirection><FeatureName></FeatureName></SecondaryAxis></Value></Frame></Frames>  GraphicType=FromGeometry  MarkerShape=Sphere  MarkerSize=10  GraphicVisPropType=SimpleVisualProperties  GraphicDiffuseColor=[0.0 0.2 1.0]  GraphicSpecularColor=[0.5 0.5 0.5 1.0]  GraphicAmbientColor=[0.15 0.15 0.15 1.0]  GraphicEmissiveColor=[0.0 0.0 0.0 1.0]  GraphicShininess=75  GraphicOpacity=1.0
  U_Link3 : sm_lib/Body Elements/File Solid  ExtGeomFileName=..\Right_ARM\Link_3_right.stp  UnitType=Custom  ExtGeomFileUnits=mm  StepReaderType=HEX  ExportConvexHullGeometry=on  InertiaType=CalculateFromGeometry  Mass=Link3_Mass  MassUnits=g  CenterOfMass=[0 0 0]  CenterOfMassUnits=m  MomentsOfInertia=[1 1 1]  MomentsOfInertiaUnits=kg*m^2  ProductsOfInertia=[0 0 0]  ProductsOfInertiaUnits=kg*m^2  BasedOnType=Mass  Density=1000  DensityUnits=kg/m^3  DoExposeReferenceFrame=on  SerializedFrames=<Frames><Frame><Id>Frame1</Id><Value><Name>Mount_F</Name><Origin><Source>ReferenceFrame</Source><FeatureName></FeatureName></Origin><PrimaryAxis><DefinedDirection>+Z</DefinedDirection><Source>ReferenceFrame</Source><SourceDirection>+Z</SourceDirection><FeatureName></FeatureName></PrimaryAxis><SecondaryAxis><DefinedDirection>+X</DefinedDirection><Source>ReferenceFrame</Source><SourceDirection>+X</SourceDirection><FeatureName></FeatureName></SecondaryAxis></Value></Frame><Frame><Id>Frame2</Id><Value><Name>Joint_F</Name><Origin><Source>CenterOfMassFrame</Source><FeatureName></FeatureName></Origin><PrimaryAxis><DefinedDirection>+Z</DefinedDirection><Source>ReferenceFrame</Source><SourceDirection>+Z</SourceDirection><FeatureName></FeatureName></PrimaryAxis><SecondaryAxis><DefinedDirection>+X</DefinedDirection><Source>ReferenceFrame</Source><SourceDirection>+X</SourceDirection><FeatureName></FeatureName></SecondaryAxis></Value></Frame></Frames>  GraphicType=FromGeometry  MarkerShape=Sphere  MarkerSize=10  GraphicVisPropType=SimpleVisualProperties  GraphicDiffuseColor=[0.0 0.2 1.0]  GraphicSpecularColor=[0.5 0.5 0.5 1.0]  GraphicAmbientColor=[0.15 0.15 0.15 1.0]  GraphicEmissiveColor=[0.0 0.0 0.0 1.0]  GraphicShininess=75  GraphicOpacity=1.0
  VC_PID1 : Constant  Value=ARM_V_PID
  VC_PID2 : Constant  Value=ARM_V_PID
  VC_PID3 : Constant  Value=ARM_V_PID
  Up_ARM_Mount : PMIOPort  Side=Left
  Body_CoM : PMIOPort  Port=2  Side=Left
  ARM_BODY_Contact : PMIOPort  Port=3  Side=Left
  ARM_TARGET_Contact : PMIOPort  Port=4  Side=Left
  tag scope: Up_ARM_J=global, Up_ARM_J_Acc_Mount=global, Up_ARM_J_Acc_SB=global, Up_ARM_J_Pos_Mount=global, Up_ARM_J_Pos_SB=global, Up_ARM_J_Vel_Mount=global, Up_ARM_J_Vel_SB=global, Up_ARM_Jd=global, Up_ARM_Jdd=global, Up_ARM_Jt=global, Up_ARM_Link_Contact_flg=global
  wires:
  MATLAB Function2/1(t_cmd) -> Gain1/1
  [ARM_Jd2] -> MATLAB Function6/5(v_mea)
  Integrator1/1 -> MATLAB Function3/1(v_sig)
  MATLAB Function5/2(vd_out) -> Simulink-PS Converter1/3
  [EE_Vel] -> Reshape11/1
  Transfer Fcn1/1 -> MATLAB Function3/2(vd_sig), Integrator1/1
  Mux3/1 -> Reshape3/1
  TC_PID1/1 -> MATLAB Function4/8(tc_gain)
  Constant2/1 -> MATLAB Function2/11(dt)
  [ARM_Jd1] -> MATLAB Function4/5(v_mea)
  [Joint2_Vel] -> Reshape10/1
  PS-Simulink Converter1/1 -> [ARM_Jdd0]
  Transfer Fcn2/1 -> MATLAB Function3/3(t_mea)
  Demux/1 -> Derivative1/1, MATLAB Function2/1(cmd)
  PC_PID2/1 -> MATLAB Function6/10(pc_gain)
  [Joint2_Pos] -> Reshape6/1
  Matrix Concatenate/1 -> [Up_ARM_J_Pos_Mount]
  [ARM_J0] -> MATLAB Function2/6(p_mea)
  [ARM_J0] -> Mux/1
  [ARM_Jt0] -> Transfer Fcn9/1
  [Joint1_Vel] -> Reshape9/1
  PS-Simulink Converter21/1 -> [EE_Vel]
  Transfer Fcn4/1 -> MATLAB Function5/3(t_mea)
  Demux/2 -> MATLAB Function4/1(cmd), Derivative2/1
  [ARM_Jt2] -> Transfer Fcn6/1
  Reshape2/1 -> [Up_ARM_Jdd]
  [ARM_Jt1] -> Transfer Fcn7/1
  Transfer Fcn3/1 -> Gain/1
  PS-Simulink Converter10/1 -> [ARM_Jd2]
  MATLAB Function6/1(t_cmd) -> Scope15/1, Transfer Fcn5/1
  TC_PID3/1 -> MATLAB Function2/8(tc_gain)
  PS-Simulink Converter20/1 -> [EE_Acc]
  Gain1/1 -> Transfer Fcn1/1, Scope13/1
  [ARM_J1] -> MATLAB Function4/6(p_mea)
  [ARM_Jt1] -> MATLAB Function4/3(t_mea)
  MATLAB Function3/2(vd_out) -> Simulink-PS Converter9/3
  PS-Simulink Converter5/1 -> [ARM_Jdd1]
  Matrix Concatenate2/1 -> [Up_ARM_J_Acc_Mount]
  Integrator2/1 -> Simulink-PS Converter1/1
  PS-Simulink Converter14/1 -> [Joint1_Acc]
  [ARM_Jt0] -> Transfer Fcn2/1
  PC_PID3/1 -> MATLAB Function2/10(pc_gain)
  Mux/1 -> Reshape/1
  [ARM_Jdd1] -> Mux2/2
  Integrator3/1 -> MATLAB Function5/1(v_sig)
  MATLAB Function5/1(v_out) -> Simulink-PS Converter1/2, Integrator2/1
  Constant10/1 -> MATLAB Function6/11(dt)
  [ARM_Jt2] -> MATLAB Function6/3(t_mea)
  [ARM_Jt0] -> MATLAB Function2/3(t_mea)
  Transfer Fcn6/1 -> MATLAB Function7/3(t_mea)
  PS-Simulink Converter11/1 -> [ARM_J2]
  PS-Simulink Converter18/1 -> [Joint2_Vel]
  PS-Simulink Converter13/1 -> [Joint1_Pos]
  MATLAB Function7/1(v_out) -> Simulink-PS Converter2/2, Integrator4/1
  PS-Simulink Converter15/1 -> [Joint1_Vel]
  [Joint1_Pos] -> Reshape5/1
  PS-Simulink Converter9/1 -> [ARM_Jdd2]
  PS-Simulink Converter16/1 -> [Joint2_Pos]
  VC_PID1/1 -> MATLAB Function4/9(vc_gain)
  TC_PID2/1 -> MATLAB Function6/8(tc_gain)
  [ARM_Jdd1] -> MATLAB Function4/4(vd_mea)
  Integrator5/1 -> MATLAB Function7/1(v_sig)
  [EE_Pos] -> Reshape7/1
  Derivative2/1 -> MATLAB Function4/2(cmd_d)
  [ARM_J2] -> Mux/3
  Matrix Concatenate1/1 -> [Up_ARM_J_Vel_Mount]
  PS-Simulink Converter6/1 -> [ARM_Jd1]
  Reshape1/1 -> [Up_ARM_Jd]
  Mux1/1 -> Reshape1/1
  MATLAB Function4/1(t_cmd) -> Scope11/1, Transfer Fcn3/1
  PC_PID1/1 -> MATLAB Function4/10(pc_gain)
  Constant9/1 -> MATLAB Function4/11(dt)
  MATLAB Function7/2(vd_out) -> Simulink-PS Converter2/3
  [ARM_Jd0] -> Mux1/1
  [ARM_Jd0] -> MATLAB Function2/5(v_mea)
  VC_PID2/1 -> MATLAB Function6/9(vc_gain)
  [ARM_Jt1] -> Transfer Fcn4/1
  PS-Simulink Converter7/1 -> [ARM_J1]
  Demux/3 -> MATLAB Function6/1(cmd), Derivative3/1
  Derivative1/1 -> MATLAB Function2/2(cmd_d)
  PS-Simulink Converter2/1 -> [ARM_Jd0]
  [ARM_Jd2] -> Mux1/3
  Integrator/1 -> Simulink-PS Converter9/1
  Transfer Fcn5/1 -> Gain2/1
  [ARM_Jdd2] -> Mux2/3
  Gain2/1 -> Saturation1/1
  Derivative3/1 -> MATLAB Function6/2(cmd_d)
  PS-Simulink Converter3/1 -> [ARM_J0]
  PS-Simulink Converter17/1 -> [Joint2_Acc]
  Mux2/1 -> Reshape2/1
  Integrator4/1 -> Simulink-PS Converter2/1
  [ARM_Jdd0] -> Mux2/1
  [ARM_J1] -> Mux/2
  MATLAB Function3/1(v_out) -> Integrator/1, Simulink-PS Converter9/2
  [ARM_J2] -> MATLAB Function6/6(p_mea)
  Gain/1 -> Saturation/1
  [ARM_Jt2] -> Transfer Fcn8/1
  [ARM_Jdd2] -> MATLAB Function6/4(vd_mea)
  [ARM_Jd1] -> Mux1/2
  Reshape3/1 -> [Up_ARM_Jt]
  Reshape/1 -> Display3/1, [Up_ARM_J]
  [ARM_Jdd0] -> MATLAB Function2/4(vd_mea)
  PS-Simulink Converter19/1 -> [EE_Pos]
  VC_PID3/1 -> MATLAB Function2/9(vc_gain)
  J_cmd/1 -> [J_CMD]
  Mode/1 -> [Mode]
  [J_CMD] -> Demux/1
  Demux1/1 -> MATLAB Function2/7(mode)
  [Mode] -> Demux1/1
  Demux1/2 -> MATLAB Function4/7(mode)
  Demux1/3 -> MATLAB Function6/7(mode)
  Saturation/1 -> MATLAB Function5/2(vd_sig), Integrator3/1
  Saturation1/1 -> Integrator5/1, MATLAB Function7/2(vd_sig)
  Joint_Pos_init/1 -> Reshape4/1
  Joint0_Vel_init/1 -> Reshape8/1
  [EE_Acc] -> Reshape15/1
  [Joint2_Acc] -> Reshape14/1
  [Joint1_Acc] -> Reshape13/1
  Joint0_Acc_init/1 -> Reshape12/1
  PS-Simulink Converter25/1 -> [EE_Vel_SB]
  PS-Simulink Converter23/1 -> [EE_Pos_SB]
  PS-Simulink Converter24/1 -> [EE_Acc_SB]
  PS-Simulink Converter26/1 -> [Joint2_Acc_SB]
  PS-Simulink Converter22/1 -> [Joint2_Pos_SB]
  PS-Simulink Converter27/1 -> [Joint2_Vel_SB]
  PS-Simulink Converter29/1 -> [Joint1_Acc_SB]
  PS-Simulink Converter28/1 -> [Joint1_Pos_SB]
  PS-Simulink Converter30/1 -> [Joint1_Vel_SB]
  PS-Simulink Converter32/1 -> [Joint0_Acc_SB]
  PS-Simulink Converter33/1 -> [Joint0_Vel_SB]
  PS-Simulink Converter31/1 -> [Joint0_Pos_SB]
  [EE_Pos_SB] -> Reshape19/1
  Matrix Concatenate3/1 -> [Up_ARM_J_Pos_SB]
  [Joint2_Pos_SB] -> Reshape18/1
  [Joint1_Pos_SB] -> Reshape17/1
  [Joint0_Pos_SB] -> Reshape16/1
  [Joint2_Vel_SB] -> Reshape22/1
  [EE_Vel_SB] -> Reshape23/1
  Matrix Concatenate4/1 -> [Up_ARM_J_Vel_SB]
  [Joint1_Vel_SB] -> Reshape21/1
  [Joint0_Vel_SB] -> Reshape20/1
  [Joint1_Acc_SB] -> Reshape25/1
  [Joint2_Acc_SB] -> Reshape26/1
  [EE_Acc_SB] -> Reshape27/1
  [Joint0_Acc_SB] -> Reshape24/1
  Reshape4/1 -> Matrix Concatenate/1
  Reshape5/1 -> Matrix Concatenate/2
  Reshape6/1 -> Matrix Concatenate/3
  Reshape7/1 -> Matrix Concatenate/4
  Reshape8/1 -> Matrix Concatenate1/1
  Reshape11/1 -> Matrix Concatenate1/4
  Reshape10/1 -> Matrix Concatenate1/3
  Reshape9/1 -> Matrix Concatenate1/2
  Reshape12/1 -> Matrix Concatenate2/1
  Reshape13/1 -> Matrix Concatenate2/2
  Reshape15/1 -> Matrix Concatenate2/4
  Reshape14/1 -> Matrix Concatenate2/3
  Reshape16/1 -> Matrix Concatenate3/1
  Reshape17/1 -> Matrix Concatenate3/2
  Reshape18/1 -> Matrix Concatenate3/3
  Reshape19/1 -> Matrix Concatenate3/4
  Reshape20/1 -> Matrix Concatenate4/1
  Reshape21/1 -> Matrix Concatenate4/2
  Reshape22/1 -> Matrix Concatenate4/3
  Reshape23/1 -> Matrix Concatenate4/4
  Reshape27/1 -> Matrix Concatenate5/4
  Reshape25/1 -> Matrix Concatenate5/2
  Reshape24/1 -> Matrix Concatenate5/1
  Reshape26/1 -> Matrix Concatenate5/3
  Matrix Concatenate5/1 -> [Up_ARM_J_Acc_SB]
  PS-Simulink Converter35/1 -> [Link2_Contact_flg]
  [Link2_Contact_flg] -> Mux4/2
  [Link1_Contact_flg] -> Mux4/1
  [Link3_Contact_flg] -> Mux4/3
  Mux4/1 -> Reshape28/1
  Reshape28/1 -> [Up_ARM_Link_Contact_flg]
  PS-Simulink Converter34/1 -> [Link3_Contact_flg]
  PS-Simulink Converter36/1 -> [Link1_Contact_flg]
  PS-Simulink Converter4/1 -> [ARM_Jt0]
  PS-Simulink Converter8/1 -> [ARM_Jt1]
  PS-Simulink Converter12/1 -> [ARM_Jt2]
  Transfer Fcn9/1 -> Mux3/1
  Transfer Fcn7/1 -> Mux3/2
  Transfer Fcn8/1 -> Mux3/3
  connections:
  U_Joint2_Motor/LConn1 -- U_Joint2_Mount_Pos/RConn1
  U_Joint1_Motor/LConn2 -- U_Joint1_Motor_Pos/LConn1
  U_Joint0_Motor/LConn2 -- U_Joint0_Motor_Pos/LConn1
  Transform Sensor3/RConn2 -- PS-Simulink Converter19/LConn1
  PS-Simulink Converter11/LConn1 -- U_Joint2/RConn2
  Simulink-PS Converter1/RConn1 -- U_Joint1/LConn2
  U_Joint0_Mount_ROT/RConn1 -- U_Joint0_Motor/LConn1
  U_Joint0/RConn2 -- PS-Simulink Converter3/LConn1
  U_Joint1/RConn5 -- PS-Simulink Converter8/LConn1
  U_Joint1/RConn1 -- U_Link2/LConn1
  U_Joint1/RConn4 -- PS-Simulink Converter5/LConn1
  Spatial Contact Force/RConn1 -- U_Link3/RConn2 -- Spatial Contact Force5/LConn1
  Simulink-PS Converter2/RConn1 -- U_Joint2/LConn2
  PS-Simulink Converter2/LConn1 -- U_Joint0/RConn3
  U_Joint1_Motor/LConn1 -- U_Joint1_Mount_Pos/RConn1
  PS-Simulink Converter13/LConn1 -- Transform Sensor1/RConn2
  U_Joint1_Motor_Pos/RConn1 -- U_Joint1/LConn1 -- Transform Sensor1/RConn1 -- Transform Sensor5/RConn1
  Simulink-PS Converter9/RConn1 -- U_Joint0/LConn2
  PS-Simulink Converter1/LConn1 -- U_Joint0/RConn4
  U_Joint2/RConn5 -- PS-Simulink Converter12/LConn1
  U_Joint2/LConn1 -- U_Joint2_Motor_Pos/RConn1 -- Transform Sensor2/RConn1 -- Transform Sensor6/RConn1
  U_Joint0/RConn1 -- U_Link1/LConn1
  U_Link3/LConn1 -- U_EE/LConn1 -- U_Joint2/RConn1
  Transform Sensor3/RConn3 -- PS-Simulink Converter21/LConn1
  U_Joint0_Motor_Pos/RConn1 -- U_Joint0/LConn1 -- Transform Sensor1/LConn1 -- Transform Sensor3/LConn1 -- Transform Sensor2/LConn1 -- Transform Sensor4/RConn1
  Spatial Contact Force4/LConn1 -- ARM_TARGET_Contact/RConn1 -- Spatial Contact Force/LConn1 -- Spatial Contact Force2/LConn1
  U_Link1/LConn2 -- U_Joint1_Mount_Pos/LConn1
  Transform Sensor2/RConn4 -- PS-Simulink Converter17/LConn1
  Transform Sensor3/RConn4 -- PS-Simulink Converter20/LConn1
  U_Joint2_Motor/LConn2 -- U_Joint2_Motor_Pos/LConn1
  PS-Simulink Converter7/LConn1 -- U_Joint1/RConn2
  U_Joint2/RConn3 -- PS-Simulink Converter10/LConn1
  U_Link2/LConn2 -- U_Joint2_Mount_Pos/LConn1
  PS-Simulink Converter16/LConn1 -- Transform Sensor2/RConn2
  Transform Sensor2/RConn3 -- PS-Simulink Converter18/LConn1
  U_Joint2/RConn4 -- PS-Simulink Converter9/LConn1
  Transform Sensor1/RConn3 -- PS-Simulink Converter15/LConn1
  Transform Sensor3/RConn1 -- U_EE/RConn1 -- Transform Sensor8/RConn1
  Spatial Contact Force3/LConn1 -- U_Link1/RConn2 -- Spatial Contact Force4/RConn1
  Spatial Contact Force2/RConn1 -- U_Link2/RConn2 -- Spatial Contact Force1/LConn1
  Transform Sensor1/RConn4 -- PS-Simulink Converter14/LConn1
  U_Joint1/RConn3 -- PS-Simulink Converter6/LConn1
  Spatial Contact Force1/RConn1 -- ARM_BODY_Contact/RConn1 -- Spatial Contact Force3/RConn1 -- Spatial Contact Force5/RConn1
  U_Joint0/RConn5 -- PS-Simulink Converter4/LConn1
  Up_ARM_Mount/RConn1 -- U_Joint0_Mount_Pos/LConn1
  Transform Sensor8/LConn1 -- Transform Sensor6/LConn1 -- Transform Sensor5/LConn1 -- Body_CoM/RConn1 -- Transform Sensor4/LConn1
  PS-Simulink Converter23/LConn1 -- Transform Sensor8/RConn2
  Transform Sensor8/RConn3 -- PS-Simulink Converter25/LConn1
  Transform Sensor8/RConn4 -- PS-Simulink Converter24/LConn1
  PS-Simulink Converter22/LConn1 -- Transform Sensor6/RConn2
  Transform Sensor6/RConn3 -- PS-Simulink Converter27/LConn1
  Transform Sensor6/RConn4 -- PS-Simulink Converter26/LConn1
  PS-Simulink Converter28/LConn1 -- Transform Sensor5/RConn2
  Transform Sensor5/RConn3 -- PS-Simulink Converter30/LConn1
  Transform Sensor5/RConn4 -- PS-Simulink Converter29/LConn1
  PS-Simulink Converter31/LConn1 -- Transform Sensor4/RConn2
  Transform Sensor4/RConn4 -- PS-Simulink Converter32/LConn1
  Transform Sensor4/RConn3 -- PS-Simulink Converter33/LConn1
  Spatial Contact Force/RConn2 -- PS-Simulink Converter34/LConn1
  Spatial Contact Force2/RConn2 -- PS-Simulink Converter35/LConn1
  Spatial Contact Force4/RConn2 -- PS-Simulink Converter36/LConn1
  U_Joint0_Mount_Pos/RConn1 -- U_Joint0_Mount_ROT/LConn1
